simulink model "simulation_commande_backstepping"  (R2020a)
settings: Solver=ode23  StartTime=0.0  StopTime=100  MaxStep=0.2  RelTol=1e-3
values from neighbouring files (symbols this model uses):
  a = 1    [Adap.m]    (also in Adaptive_control_Non_linear.m = 2; HOSM.m; projet_AAV.m; sys.m)
  b = 2    [Adaptive_Control_Linear.m]    (also in Adaptive_control_Non_linear.m; HOSM.m = 1; feedback-integrator.m = 3; mini_projet.m = 3)
  lambda = 0.3    [fuzzy.m]    (also in projet_AAV.m = 1)
settings Model: Creator=lenovo  LastModifiedBy=lenovo
settings SolverCC: AlgebraicLoopSolver=LineSearch

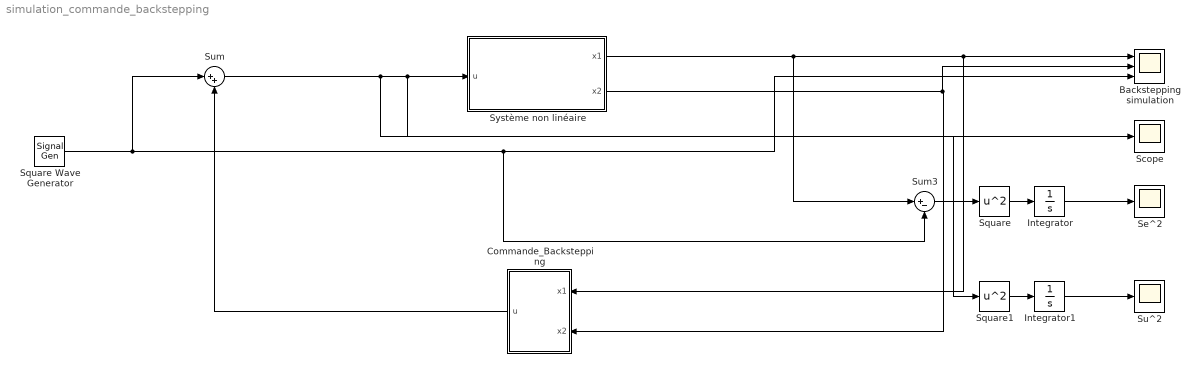
== system simulation_commande_backstepping ==
  Backstepping simulation : Scope  NumInputPorts=3
  Commande_Backstepping : Subsystem
  Integrator : Integrator
  Integrator1 : Integrator
  Scope : Scope
  Se^2 : Scope
  Square : Math  Operator=square  SaturateOnIntegerOverflow=on
  Square Wave Generator : SignalGenerator  WaveForm=square  Frequency=0.1  Units=rad/sec
  Square1 : Math  Operator=square  SaturateOnIntegerOverflow=on
  Su^2 : Scope
  Sum : Sum  Inputs=|++
  Sum3 : Sum  Inputs=|+-
  Système non linéaire : Subsystem
  wires:
  Sum/1 -> Square1/1, Scope/1, Système non linéaire/1(u)
  Commande_Backstepping/1(u) -> Sum/2
  Système non linéaire/2(x2) -> Backstepping simulation/2, Commande_Backstepping/2(x2)
  Sum3/1 -> Square/1
  Square/1 -> Integrator/1
  Integrator/1 -> Se^2/1
  Integrator1/1 -> Su^2/1
  Square1/1 -> Integrator1/1
  Système non linéaire/1(x1) -> Sum3/1, Backstepping simulation/1, Commande_Backstepping/1(x1)
  Square Wave Generator/1 -> Sum3/2, Backstepping simulation/3, Sum/1

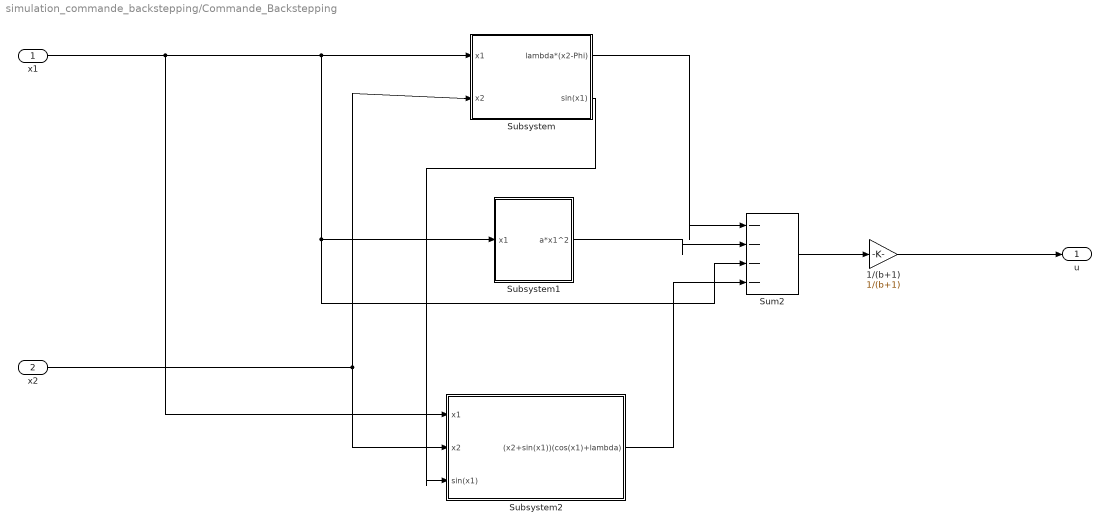
== system simulation_commande_backstepping/Commande_Backstepping ==
  x1 : Inport
  x2 : Inport  Port=2
  1/(b+1) : Gain  Gain=1/(b+1)
  Subsystem : Subsystem
  Subsystem1 : Subsystem
  Subsystem2 : Subsystem
  Sum2 : Sum  Inputs=|----
  u : Outport
  wires:
  x1/1 -> Subsystem2/1("x1 "), Subsystem/1(x1), Sum2/3, Subsystem1/1("x1 ")
  x2/1 -> Subsystem2/2(x2), Subsystem/2(x2)
  Sum2/1 -> 1/(b+1)/1
  1/(b+1)/1 -> u/1
  Subsystem/1(lambda*(x2-Phi)) -> Sum2/1
  Subsystem1/1(a*x1^2) -> Sum2/2
  Subsystem/2(sin(x1)) -> Subsystem2/3(sin(x1))
  Subsystem2/1((x2+sin(x1))(cos(x1)+lambda)) -> Sum2/4

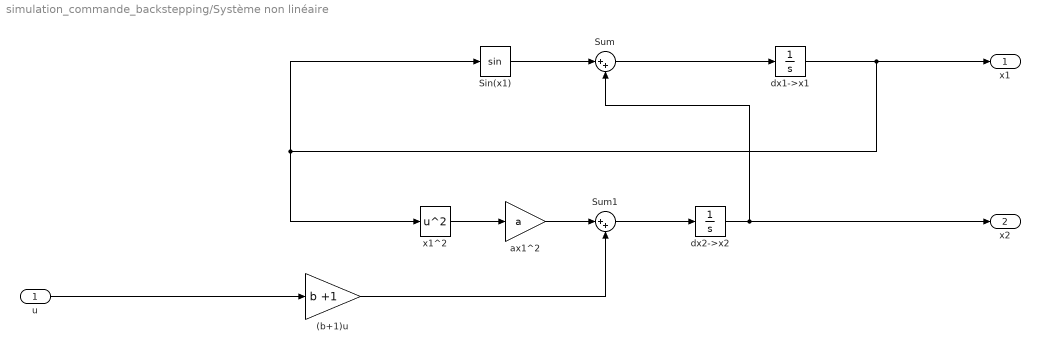
== system simulation_commande_backstepping/Système non linéaire ==
  u : Inport
  (b+1)u : Gain  Gain=b +1
  Sin(x1) : Trigonometry
  Sum : Sum  Inputs=|++
  Sum1 : Sum  Inputs=|++
  ax1^2 : Gain  Gain=a
  dx1->x1 : Integrator
  dx2->x2 : Integrator
  x1^2 : Math  Operator=square  SaturateOnIntegerOverflow=on
  x1 : Outport
  x2 : Outport  Port=2
  wires:
  (b+1)u/1 -> Sum1/2
  dx2->x2/1 -> x2/1, Sum/2
  u/1 -> (b+1)u/1
  ax1^2/1 -> Sum1/1
  dx1->x1/1 -> Sin(x1)/1, x1^2/1, x1/1
  Sin(x1)/1 -> Sum/1
  x1^2/1 -> ax1^2/1
  Sum1/1 -> dx2->x2/1
  Sum/1 -> dx1->x1/1

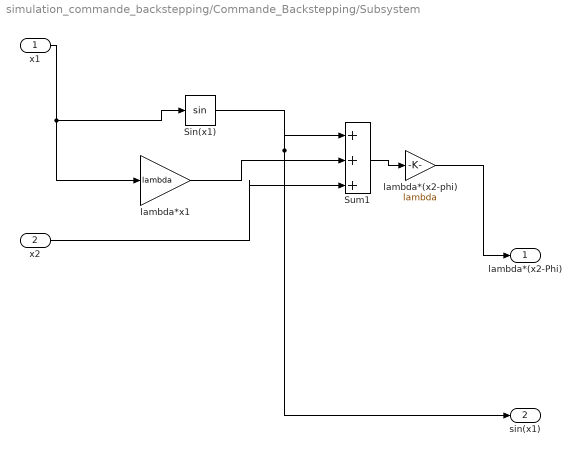
== system simulation_commande_backstepping/Commande_Backstepping/Subsystem ==
  x1 : Inport
  x2 : Inport  Port=2
  Sin(x1) : Trigonometry
  Sum1 : Sum  Inputs=|+++
  lambda*(x2-phi) : Gain  Gain=lambda
  lambda*x1 : Gain  Gain=lambda
  lambda*(x2-Phi) : Outport
  sin(x1) : Outport  Port=2
  wires:
  x1/1 -> Sin(x1)/1, lambda*x1/1
  Sin(x1)/1 -> sin(x1)/1, Sum1/1
  Sum1/1 -> lambda*(x2-phi)/1
  x2/1 -> Sum1/3
  lambda*x1/1 -> Sum1/2
  lambda*(x2-phi)/1 -> lambda*(x2-Phi)/1

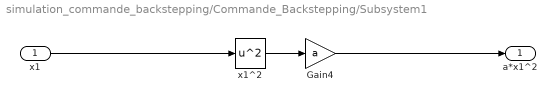
== system simulation_commande_backstepping/Commande_Backstepping/Subsystem1 ==
  "x1 " : Inport
  Gain4 : Gain  Gain=a
  x1^2 : Math  Operator=square  SaturateOnIntegerOverflow=on
  a*x1^2 : Outport
  wires:
  x1^2/1 -> Gain4/1
  Gain4/1 -> a*x1^2/1
  "x1 "/1 -> x1^2/1

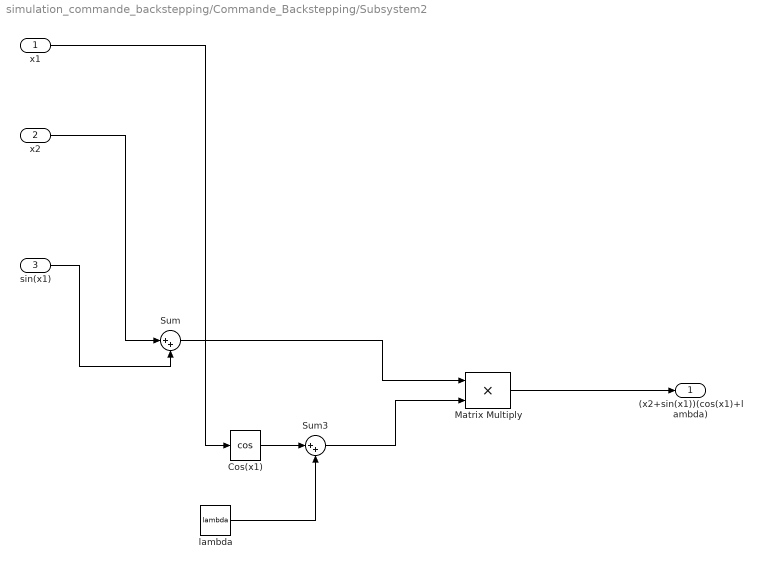
== system simulation_commande_backstepping/Commande_Backstepping/Subsystem2 ==
  "x1 " : Inport
  x2 : Inport  Port=2
  sin(x1) : Inport  Port=3
  Cos(x1) : Trigonometry  Operator=cos
  Matrix Multiply : Product
  Sum : Sum  Inputs=|++
  Sum3 : Sum  Inputs=|++
  lambda : Constant  Value=lambda  OutDataTypeStr=Inherit: Inherit via back propagation
  (x2+sin(x1))(cos(x1)+lambda) : Outport
  wires:
  Cos(x1)/1 -> Sum3/1
  sin(x1)/1 -> Sum/2
  lambda/1 -> Sum3/2
  x2/1 -> Sum/1
  Matrix Multiply/1 -> (x2+sin(x1))(cos(x1)+lambda)/1
  Sum/1 -> Matrix Multiply/1
  Sum3/1 -> Matrix Multiply/2
  "x1 "/1 -> Cos(x1)/1
